simulink model "Running_mex_SIMULINK_No_controller"  (R2020a)
settings: Solver=VariableStepAuto  StartTime=0.0  StopTime=inf  RelTol=1e-3
values from neighbouring files (symbols this model uses):
  Ctorque1 = 0/1000    (= 0)    [simulink_run_file.m]
  Ctorque2 = 0/1000    (= 0)    [simulink_run_file.m]
  Ctorque3 = 2/1000    (= 0.002)    [simulink_run_file.m]
  refresh = .02    (= 0.02)    [simulink_run_file.m]
  Tfinal_master = 1    [simulink_run_file.m]
undefined symbols (not defined in the file or in its folder): get_initial_inputs
settings Model: Creator=hoddid  LastModifiedBy=hoddid
settings DebuggingCC: UnderSpecifiedDimensionMsg=warning

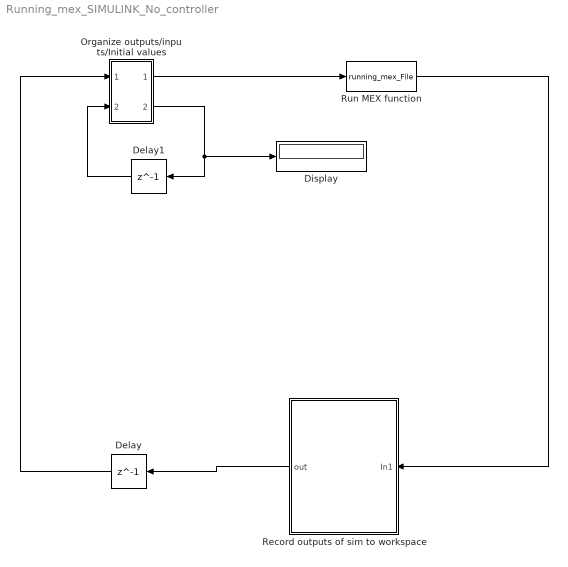
== system Running_mex_SIMULINK_No_controller ==
  Delay : Delay  DelayLength=1
  Delay1 : Delay  DelayLength=1
  Display : Display
  Organize outputs/inputs/Initial values : Subsystem
  Record outputs of sim to workspace : Subsystem
  Run MEX function : MATLABFcn  MATLABFcn=running_mex_File  OutputDimensions=[1 32]  Output1D=off
  wires:
  Run MEX function/1 -> Record outputs of sim to workspace/1(In1)
  Record outputs of sim to workspace/1(out) -> Delay/1
  Organize outputs/inputs/Initial values/1(sim_params) -> Run MEX function/1
  Delay/1 -> Organize outputs/inputs/Initial values/1(In1)
  Organize outputs/inputs/Initial values/2(Ttotal) -> Delay1/1, Display/1
  Delay1/1 -> Organize outputs/inputs/Initial values/2(In2)

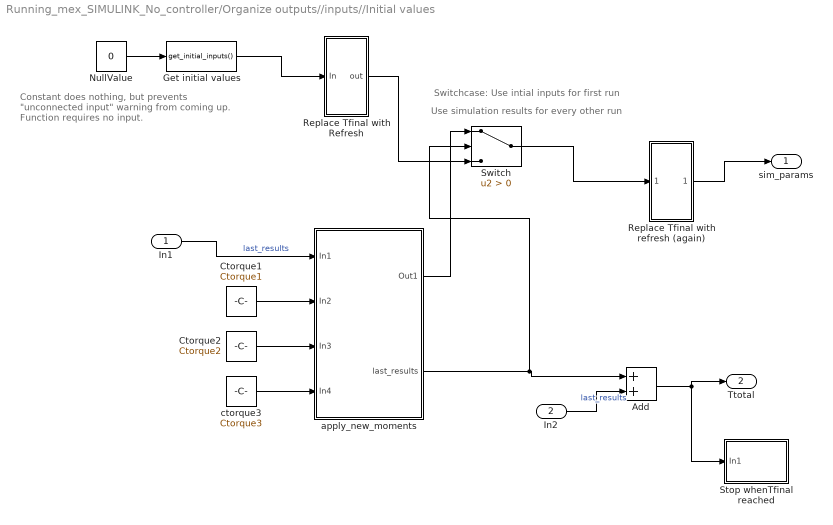
== system Running_mex_SIMULINK_No_controller/Organize outputs//inputs//Initial values ==
  note: Use simulation results for every other run
  note: Switchcase: Use intial inputs for first run
  note: Constant does nothing, but prevents
      | "unconnected input" warning from coming up.
      | Function requires no input.
  In1 : Inport
  In2 : Inport  Port=2
  Add : Sum
  Ctorque1 : Constant  Value=Ctorque1
  Ctorque2 : Constant  Value=Ctorque2
  Get initial values : MATLABFcn  MATLABFcn=get_initial_inputs()  Output1D=off
  NullValue : Constant  Value=0
  Replace Tfinal with Refresh : Subsystem
  Replace Tfinal with refresh (again) : Subsystem
  Stop whenTfinal reached : Subsystem
      settings: PortSchema="{\"entries\":[{\"content\":{\"sides\":[{\"content\":{\"connectorIds\":[]},\"type\":\"ConnectorPlacement.EquallySpacedRectSide\",\"uuid\":\"b8031d13-d17c-4f9a-b5f8-92da6927a3ba\"},{\"content\":{\"connectorIds\":[],\"side\":\"RIGHT\"},\"type\":\"ConnectorPlacement.EquallySpacedRectSide\",\"uuid\":\"11a71682-1cdb-45f2-b8b8-d175538f4c28\"},{\"content\":{\"connectorIds\":[\"In1\"],\"side\":\"TOP\"},\"type\":\"ConnectorPlacement.EquallySpacedRectSide\",\"uuid\":\"ae57efda-2ecd-443a-aa6f-cfe1c35dec26\"}]},\"type\":\"ConnectorPlacement.EquallySpacedConnector\",\"uuid\":\"64a769af-a08f-48b5-9fd8-ee733c537d04\"}],\"packageUris\":[\"http://schema.mathworks.com/mf0/Connector/19700101\"],\"version\":\"1.0\"}"
  Switch : Switch  Criteria=u2 > Threshold
  apply_new_moments : Subsystem
  ctorque3 : Constant  Value=Ctorque3
  sim_params : Outport
  Ttotal : Outport  Port=2
  wires:
  In1/1 -> apply_new_moments/1(In1)  "last_results"
  Ctorque1/1 -> apply_new_moments/2(In2)
  Ctorque2/1 -> apply_new_moments/3(In3)
  ctorque3/1 -> apply_new_moments/4(In4)
  apply_new_moments/1(Out1) -> Switch/1
  apply_new_moments/2(last_results) -> Switch/2, Add/1
  In2/1 -> Add/2  "last_results"
  Add/1 -> Ttotal/1, Stop whenTfinal reached/1(In1)
  Switch/1 -> Replace Tfinal with refresh (again)/1(In1)
  Get initial values/1 -> Replace Tfinal with Refresh/1(In)
  Replace Tfinal with Refresh/1(out) -> Switch/3
  Replace Tfinal with refresh (again)/1(last_results) -> sim_params/1
  NullValue/1 -> Get initial values/1

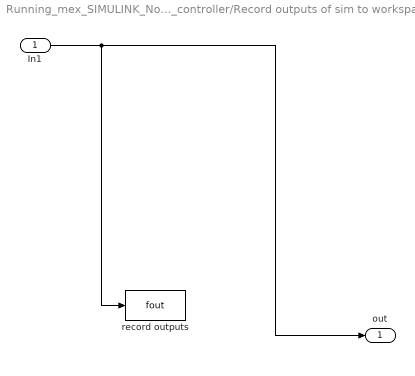
== system Running_mex_SIMULINK_No_controller/Record outputs of sim to workspace ==
  In1 : Inport
  record outputs : ToWorkspace  VariableName=fout  SampleTime=-1
      settings: Save2DSignal=2-D array (concatenate along first dimension)
  out : Outport
  wires:
  In1/1 -> out/1, record outputs/1

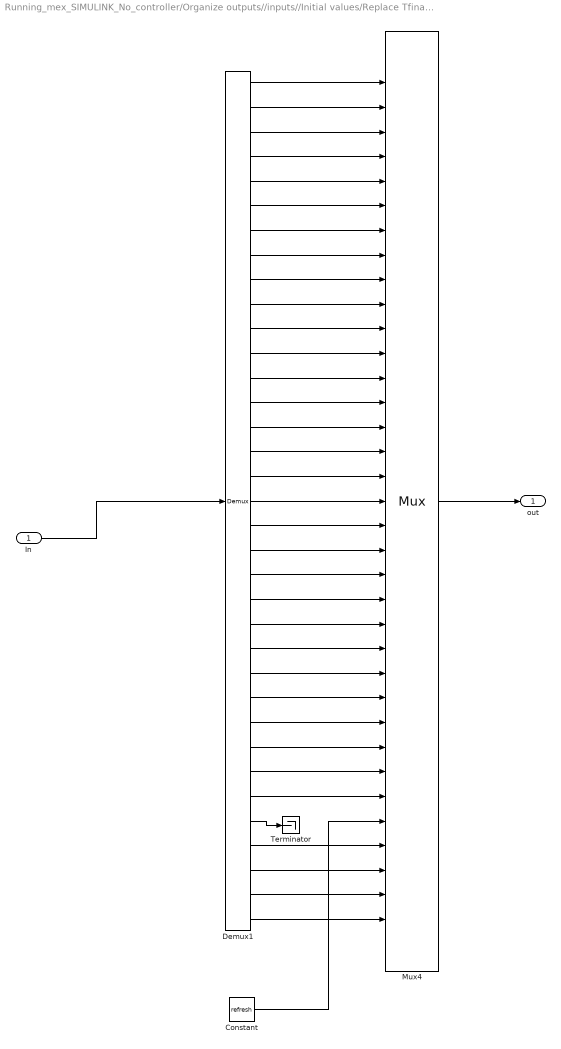
== system Running_mex_SIMULINK_No_controller/Organize outputs//inputs//Initial values/Replace Tfinal with Refresh ==
  In : Inport
  Constant : Constant  Value=refresh
  Demux1 : Demux  Outputs=35
  Mux4 : Mux  Inputs=35
  Terminator : Terminator
  out : Outport  OutDataTypeStr=double
  wires:
  In/1 -> Demux1/1
  Mux4/1 -> out/1
  Demux1/1 -> Mux4/1
  Demux1/2 -> Mux4/2
  Demux1/3 -> Mux4/3
  Demux1/4 -> Mux4/4
  Demux1/5 -> Mux4/5
  Demux1/6 -> Mux4/6
  Demux1/7 -> Mux4/7
  Demux1/8 -> Mux4/8
  Demux1/9 -> Mux4/9
  Demux1/10 -> Mux4/10
  Demux1/11 -> Mux4/11
  Demux1/12 -> Mux4/12
  Demux1/13 -> Mux4/13
  Demux1/14 -> Mux4/14
  Demux1/15 -> Mux4/15
  Demux1/16 -> Mux4/16
  Demux1/17 -> Mux4/17
  Demux1/18 -> Mux4/18
  Demux1/19 -> Mux4/19
  Demux1/20 -> Mux4/20
  Demux1/21 -> Mux4/21
  Demux1/22 -> Mux4/22
  Demux1/23 -> Mux4/23
  Demux1/24 -> Mux4/24
  Demux1/25 -> Mux4/25
  Demux1/26 -> Mux4/26
  Demux1/27 -> Mux4/27
  Demux1/28 -> Mux4/28
  Demux1/29 -> Mux4/29
  Constant/1 -> Mux4/31
  Demux1/31 -> Terminator/1
  Demux1/35 -> Mux4/35
  Demux1/34 -> Mux4/34
  Demux1/33 -> Mux4/33
  Demux1/32 -> Mux4/32
  Demux1/30 -> Mux4/30

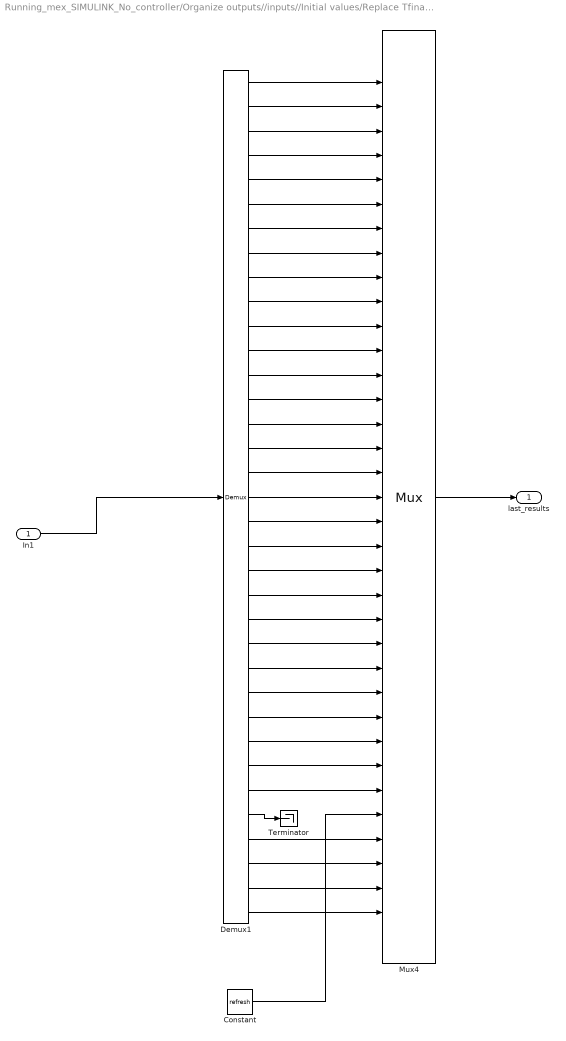
== system Running_mex_SIMULINK_No_controller/Organize outputs//inputs//Initial values/Replace Tfinal with refresh (again) ==
  In1 : Inport
  Constant : Constant  Value=refresh
  Demux1 : Demux  Outputs=35
  Mux4 : Mux  Inputs=35
  Terminator : Terminator
  last_results : Outport  OutDataTypeStr=double
  wires:
  In1/1 -> Demux1/1
  Mux4/1 -> last_results/1
  Demux1/1 -> Mux4/1
  Demux1/2 -> Mux4/2
  Demux1/3 -> Mux4/3
  Demux1/4 -> Mux4/4
  Demux1/5 -> Mux4/5
  Demux1/6 -> Mux4/6
  Demux1/7 -> Mux4/7
  Demux1/8 -> Mux4/8
  Demux1/9 -> Mux4/9
  Demux1/10 -> Mux4/10
  Demux1/11 -> Mux4/11
  Demux1/12 -> Mux4/12
  Demux1/13 -> Mux4/13
  Demux1/14 -> Mux4/14
  Demux1/15 -> Mux4/15
  Demux1/16 -> Mux4/16
  Demux1/17 -> Mux4/17
  Demux1/18 -> Mux4/18
  Demux1/19 -> Mux4/19
  Demux1/20 -> Mux4/20
  Demux1/21 -> Mux4/21
  Demux1/22 -> Mux4/22
  Demux1/23 -> Mux4/23
  Demux1/24 -> Mux4/24
  Demux1/25 -> Mux4/25
  Demux1/26 -> Mux4/26
  Demux1/27 -> Mux4/27
  Demux1/28 -> Mux4/28
  Demux1/29 -> Mux4/29
  Constant/1 -> Mux4/31
  Demux1/31 -> Terminator/1
  Demux1/35 -> Mux4/35
  Demux1/34 -> Mux4/34
  Demux1/33 -> Mux4/33
  Demux1/32 -> Mux4/32
  Demux1/30 -> Mux4/30

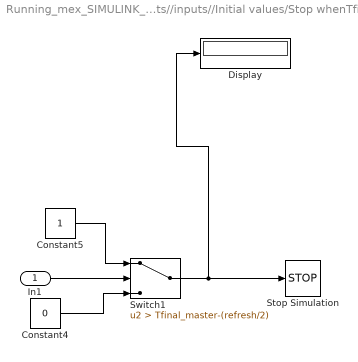
== system Running_mex_SIMULINK_No_controller/Organize outputs//inputs//Initial values/Stop whenTfinal reached ==
  In1 : Inport
  Constant4 : Constant  Value=0
  Constant5 : Constant
  Display : Display
  Stop Simulation : Stop
  Switch1 : Switch  Criteria=u2 > Threshold  Threshold=Tfinal_master-(refresh/2)
  wires:
  Constant4/1 -> Switch1/3
  In1/1 -> Switch1/2
  Switch1/1 -> Display/1, Stop Simulation/1
  Constant5/1 -> Switch1/1

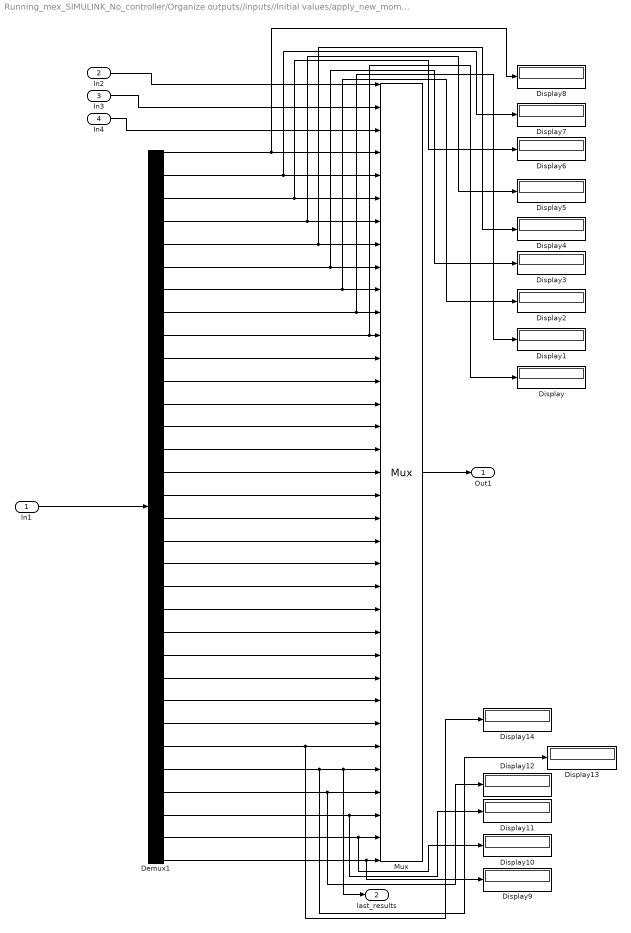
== system Running_mex_SIMULINK_No_controller/Organize outputs//inputs//Initial values/apply_new_moments ==
  In1 : Inport
  In2 : Inport  Port=2
  In3 : Inport  Port=3
  In4 : Inport  Port=4
  Demux1 : Demux  Outputs=32
  Display{,1..14} (15 alike) : Display
  Mux : Mux  Inputs=35
  Out1 : Outport  OutDataTypeStr=double
  last_results : Outport  Port=2
  wires:
  In1/1 -> Demux1/1
  In4/1 -> Mux/3
  In3/1 -> Mux/2
  In2/1 -> Mux/1
  Mux/1 -> Out1/1
  Demux1/1 -> Display8/1, Mux/4
  Demux1/2 -> Display7/1, Mux/5
  Demux1/3 -> Display6/1, Mux/6
  Demux1/4 -> Display5/1, Mux/7
  Demux1/5 -> Display4/1, Mux/8
  Demux1/6 -> Display3/1, Mux/9
  Demux1/7 -> Display2/1, Mux/10
  Demux1/8 -> Display1/1, Mux/11
  Demux1/9 -> Display/1, Mux/12
  Demux1/10 -> Mux/13
  Demux1/11 -> Mux/14
  Demux1/12 -> Mux/15
  Demux1/13 -> Mux/16
  Demux1/14 -> Mux/17
  Demux1/15 -> Mux/18
  Demux1/16 -> Mux/19
  Demux1/17 -> Mux/20
  Demux1/18 -> Mux/21
  Demux1/19 -> Mux/22
  Demux1/20 -> Mux/23
  Demux1/21 -> Mux/24
  Demux1/22 -> Mux/25
  Demux1/23 -> Mux/26
  Demux1/24 -> Mux/27
  Demux1/25 -> Mux/28
  Demux1/26 -> Mux/29
  Demux1/27 -> Display14/1, Mux/30
  Demux1/28 -> Display13/1, last_results/1, Mux/31
  Demux1/29 -> Mux/32, Display12/1
  Demux1/30 -> Display11/1, Mux/33
  Demux1/31 -> Display10/1, Mux/34
  Demux1/32 -> Display9/1, Mux/35
